simulink model "TwoBeamSEb"  (R2015b)
settings: Solver=VariableStepAuto  StartTime=0.0  StopTime=10.0  RelTol=1e-3
undefined symbols (not defined in the file or in its folder): c2
libraries: cstblocks x2
settings Model: Creator=d.alazard  LastModifiedBy=d.alazard

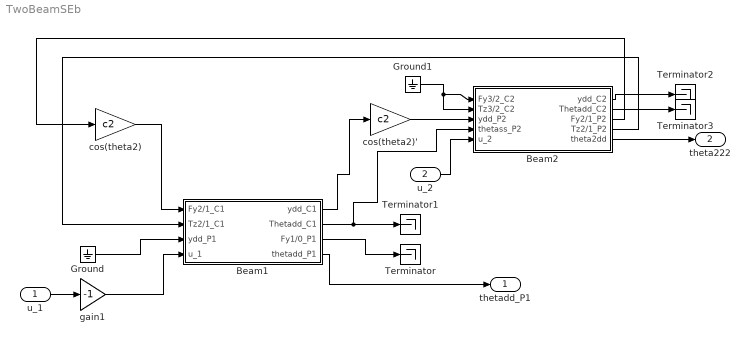
== system TwoBeamSEb ==
  u_1 : Inport
  u_2 : Inport  Port=2
  Beam1 : Subsystem
  Beam2 : Subsystem
  Ground : Ground
  Ground1 : Ground
  Terminator{,1..3} (4 alike) : Terminator
  cos(theta2) : Gain  Gain=c2
  cos(theta2)' : Gain  Gain=c2
  gain1 : Gain  Gain=-1
  thetadd_P1 : Outport
  theta222 : Outport  Port=2
  wires:
  u_1/1 -> gain1/1
  Beam1/3(Fy1/0_P1) -> Terminator/1
  Beam1/4(thetadd_P1) -> thetadd_P1/1
  Ground/1 -> Beam1/3(ydd_P1)
  Beam1/2(Thetadd_C1) -> Beam2/4(thetass_P2), Terminator1/1
  Beam1/1(ydd_C1) -> cos(theta2)'/1
  cos(theta2)'/1 -> Beam2/3(ydd_P2)
  cos(theta2)/1 -> Beam1/1(Fy2/1_C1)
  Beam2/3(Fy2/1_P2) -> cos(theta2)/1
  Ground1/1 -> Beam2/1(Fy3/2_C2), Beam2/2(Tz3/2_C2)
  Beam2/2(Thetadd_C2) -> Terminator3/1
  Beam2/1(ydd_C2) -> Terminator2/1
  gain1/1 -> Beam1/4(u_1)
  u_2/1 -> Beam2/5(u_2)
  Beam2/5(theta2dd) -> theta222/1
  Beam2/4(Tz2/1_P2) -> Beam1/2(Tz2/1_C1)

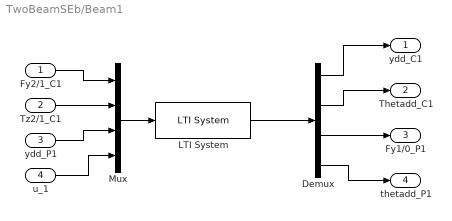
== system TwoBeamSEb/Beam1 ==
  Fy2/1_C1 : Inport
  Tz2/1_C1 : Inport  Port=2
  ydd_P1 : Inport  Port=3
  u_1 : Inport  Port=4
  Demux : Demux
  LTI System : cstblocks/LTI System  sys=Mm1_4  IC=[]
  Mux : Mux
  ydd_C1 : Outport
  Thetadd_C1 : Outport  Port=2
  Fy1/0_P1 : Outport  Port=3
  thetadd_P1 : Outport  Port=4
  wires:
  LTI System/1 -> Demux/1
  Demux/4 -> thetadd_P1/1
  ydd_P1/1 -> Mux/3
  Fy2/1_C1/1 -> Mux/1
  Tz2/1_C1/1 -> Mux/2
  u_1/1 -> Mux/4
  Demux/1 -> ydd_C1/1
  Demux/2 -> Thetadd_C1/1
  Demux/3 -> Fy1/0_P1/1
  Mux/1 -> LTI System/1

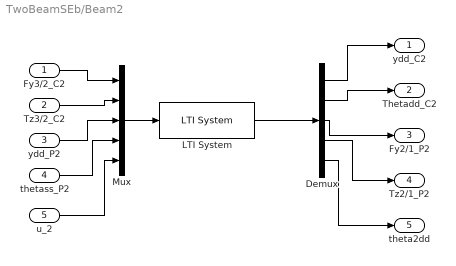
== system TwoBeamSEb/Beam2 ==
  Fy3/2_C2 : Inport
  Tz3/2_C2 : Inport  Port=2
  ydd_P2 : Inport  Port=3
  thetass_P2 : Inport  Port=4
  u_2 : Inport  Port=5
  Demux : Demux  Outputs=5
  LTI System : cstblocks/LTI System  sys=M2am1_5  IC=[]
  Mux : Mux  Inputs=5
  ydd_C2 : Outport
  Thetadd_C2 : Outport  Port=2
  Fy2/1_P2 : Outport  Port=3
  Tz2/1_P2 : Outport  Port=4
  theta2dd : Outport  Port=5
  wires:
  Mux/1 -> LTI System/1
  Demux/3 -> Fy2/1_P2/1
  Demux/2 -> Thetadd_C2/1
  Demux/1 -> ydd_C2/1
  thetass_P2/1 -> Mux/4
  Tz3/2_C2/1 -> Mux/2
  Fy3/2_C2/1 -> Mux/1
  ydd_P2/1 -> Mux/3
  Demux/4 -> Tz2/1_P2/1
  LTI System/1 -> Demux/1
  Demux/5 -> theta2dd/1
  u_2/1 -> Mux/5
